simulink library "DiSC_ToolboxOpal_V12"  (R2012b)
settings: Solver=ode45  StartTime=0.0  StopTime=10.0  RelTol=1e-3
undefined symbols (not defined in the file or in its folder): SamplingTime
(part 4 of 5)

== matlab function DiSC_ToolboxOpal_V12/SuperMarket/MATLAB Function ==
  data: exeDefrost input; p output; pRS input; t input; q output; timeReady output; timeDefrost output
function [p,q,timeReady,timeDefrost] = smAssetDO(exeDefrost,pRS, t)
%#codegen
% Simulink version of supermarket model using embedded MATLAB function
%%Supermarket with flexible defrost cycles for demand response purpose
%   This class implements a model of a supermarket with flexible
%   defrost cycles. The defrost cycles of low temperature display cases
%   are allowed to be shifted in time under certain bounds. The reason
%   for only using low temperature dispaly cases is that these use
%   electrical heating elements for actively melting the ice during
%   defrost cycles. These heating elements consume a substantial amount
%   of power.
%
%   For a formal description of supermarket defrost flexibility, see the
%   note on the homepage:
%   http://kom.aau.dk/project/SmartGridControl/DiSC/documentation.html
%
% Revision:
% 16-07-2014, R. Pedersen, Aalborg University. Notes:
% 29-11-2014, R. Olsen/M. Kemal, Aalborg University (Simulink)
% 20-06-2015, F. Iov/M. Kemal, Aalborg University (Simulink toolbox for OPAL)

            % Implement algorithm. Calculate y as a function of
            % input u and discrete states.
             % Input:
            %   - exeDefrost [-], is the external control signal to execute defrost cycles.
            %   - pRS [W], is the power consumption of the refrigeration system, this should be provided as data.
            %
            % Output:
            %   - p [W], is the active power consumption of the supermarket.
            %   - q [VAR], is the reactive power consumption of the supermarket.
            %   - timeReady [s], is the time until defrost cycles are ready to be executed.
            %   - timeDefrost [s], is the time until the defrost cycles will be executed by the supermarket.
            
            % Power and time flexibility from defrost cycle


    % parameter properties
        param.sBase = 3e6;            % Complex power base [VA]. 
        param.Ts = 1;                 % Sampling time [sec]. 
        param.onPU = false;           % Indicates if the supermarket is used to simulate a system on per unit basis. true = yes, false = no [-]. 
        param.numDF = 2;              % Number of low temperature display cases [-]. 
        param.PF = 0.95;              % Power factor [-].
        param.pDefrost=[3e3 10e3];    % Vector containing defrost power consumption [W]. 
        
     persistent var;
     if isempty(var) 
        var.p_c=0;      %All used for caching in between sampling period
        var.q_c=0;
        var.tr_c=zeros(2,1);
        var.tdf_c=zeros(2,1);
        var.t_c=0;         
         
         
        var.readyTimers = zeros(2,1);
        var.defrostTimers = zeros(2,1);
        var.waitTimers = ones(2,1)*60*60*3;
        
        var.timeReady=zeros(2,1);  
        var.timeDefrost=zeros(2,1);
        var.waitGuards = ones(2,1)*60*60*10;      
        var.states = ones(2,1)*2;               
        var.readyGuards = ones(2,1)*60*60*2;    
        var.defrostGuards = ones(2,1)*45*60;    
        var.pVec =zeros(2,1);           
     end    
     
     %implement algorithm
            if (param.Ts>0)
               if (t>(var.t_c+param.Ts))
                   [p,q,timeReady,timeDefrost,varNew] = sampleSM(param,var,exeDefrost,pRS);
                   var=varNew;
                   var.p_c=p;
                   var.q_c=q;
                   var.tr_c=timeReady;
                   var.tdf_c=timeDefrost;
                   var.t_c=t;
               end
               p=var.p_c;
               q=var.q_c;
               timeReady=var.tr_c;
               timeDefrost=var.tdf_c;               
            else
                [p,q,timeReady,timeDefrost,varNew] = sampleSM(param,var,exeDefrost,pRS);
                var= varNew;
            end

end

== matlab function DiSC_ToolboxOpal_V12/Tap Changer/MATLAB Function ==
  data: y1 output; vMeas input; vRef input; uRef input; mode input; day input; y2 output; y3 output; time input
function [y1,y2,y3] = tcAssetDO(vMeas,vRef,uRef,mode,day,time)
%#codegen
   %tcAssetDO implements a controllable tap changing transformer using
   %MATLAB embedded block of simulink 
   %
   %
    %   The tcAsset can change the tap position of a transformer and 
    %   thereby effectively change the transformers ratio.
    %   The tap changer can be used to simulate e.g., an on-load tap changing
    %   transformer. The tap changer works by altering the grid admittance
    %   matrix, when ever the tap position is changed. To ensure realistic
    %   simulation scenarios a minimum time between tap changes has been
    %   incorporated, along with a specified maximum number of tap changes
    %   per day.
    %   
    %   The model is intended for studing voltage control problems and can
    %   be set to run in two different modes; follow tap reference and
    %   apply voltage control. The model is based on the one found in "Power Systems
    %   Stability and Control, P. Kundur".
    %
    % Revision:
    % 03-09-2014, R. Pedersen, Aalborg University. Notes:
    % 29-11-2014, R. Olsen/M. Kemal, Aalborg University (Simulink)
    % 20-06-2015, F. Iov/M. Kemal, Aalborg University (Simulink toolbox for OPAL)
            % Input:
            %   - v, is the voltage at the connection point.
            %   - vRef, is the voltage reference for the voltage
            %     control.
            %   - uRef, is the reference to tap position.
            %   - k, is the sample.
            %   - day, is the day of the simulation (1-365).
            % 
            % Output:
            %   - y1, y2, y3, is the transformer admittances between busses,
            %     from ground to primary side bus and from ground to
            %     secondary side bus, respectively.    
    %parameter properties
        param.vBase = 20e3;               % Voltage base [V].
        param.Z = 0.03-0.13i;             % Trafo impedance [Ohm].
        param.Ts = 1;                     % Sampling time [sec].
        param.nomTapRatio = 3;            % Nominal transformer ratio [-].
        param.nTapUp = 5;                 % Number of tap position upwards [-].
        param.nTapDown = -5;              % Number of tap positions downwards [-].
        param.nTapPrDay = 10;             % Maximum number of tap changes per day [-].
        param.chPrTap = 0.0125;           % Ratio of change from nominal voltage per tap position on a per unit basis [-].
        param.tMin = 5*60;                % Minimum time between tap changes [sec]. 

    %variable properties     
     persistent var;
     if isempty(var) 
        % Setup the buffer for the moving average filter
        %vAvgFilterTemp=1;
        var.avgFilterBuf = ones(10,1);  %TODO: This has been static defined due to Simulink
        var.kMin=0 ;                       % [-]. Minimum number of samples between tap changes
        
        var.tapChOk = 0;                % [-]. Flag indicating if tap change is allowed (1=yes, 0=no) 
        var.y1 = complex(0);            % [S]. Admittance of trafo between busses
        var.y2 = complex(0);            % [S]. Admittance from ground to trafo, primary side
        var.y3 = complex(0);            % [S]. Admittance from ground to trafo, secondary side
        var.tapPos = -1;                % [-]. Tap position
        var.dayOld = -1;                % [-]. Used to check if day has changed
        var.tapChDay = 0;               % [-]. Number of tap changes that has occured in a day
        var.tapTimer = 0;               % [-]. Timer indicating if tap changing is allowed, i.e., the timer must be greater than kMin to do tap changing
        var.vHyst = 0.05;               % [%]. Hysterisis limit for voltage control
        var.avgFilterTime = 10*60;      % [s]. Time window of the moving average filter
        var.mode = 0;                   % [-]. Mode of the tap position control (0=follow tap reference, 1=voltage control
        var.t_c=0;                      % [s]. Caching time
        var.y1_c=complex(0);            % Cached y1 value
        var.y2_c=complex(0);
        var.y3_c=complex(0);
        var.k=0;                        % Sample nr.         
     end
            % Compute minimum samples between tap changes
            var.kMin = ceil(param.tMin/param.Ts);
            
            % Change the admittances of the trafo
            [var.y1_c,var.y2_c,var.y3_c] = sampletcAsset(param,var,1,1,0,1,1);
            var.tapTimer = 0;
            var.tapChDay = 0;
            var.tapChOk = 0;
            %changeTrafoAdm(obj); 
            
            % Set average filter buffer
            var.avgFilterBuf = var.avgFilterBuf*param.vBase;
            
                        % Implement algorithm. 
           
             if (param.Ts>0)
               if (time>(var.t_c+param.Ts))
                   [y1,y2,y3,varNew] = sampletcAsset(param,var,vMeas,vRef,uRef,var.k,day);
                   var=varNew;
                   var.y1_c=y1;
                   var.y2_c=y2;
                   var.y3_c=y3;
                   var.t_c=time;
                   var.k=var.k+1;
                   var.mode = mode;
               end
               y1=var.y1_c;
               y2=var.y2_c;
               y3=var.y3_c;               
            else
                [y1,y2,y3,varNew] = sampletcAsset(param,var,vMeas,vRef,uRef,var.k,day);
                var=varNew;
                var.k=var.k+1; 
             end     
                
end

== matlab function DiSC_ToolboxOpal_V12/SolarPowerPlantDO/pvAssetDO/MATLAB Function1 ==
  data: solarIrr input; p output; vMeas input; time input; dP input; dPlim input; qRef input; qMode input; vRef input; q output; pAva output
function [p,q,pAva] = pvAssetDO(solarIrr,vMeas,time,dP,dPlim,qRef,qMode,vRef)

%#codegen
%pvAssetDO implements a simple P,Q controllable solar PV system using MATLAB embedded function.
    %   The pvAsset can be set to follow an active power reference, output
    %   maximum power available or derate power. It can also, at the same
    %   time be set to follow a reactive power reference, output the
    %   minimum reactive power according to the power factor or try to keep
    %   a voltage reference in the coupling point by controlling reactive
    %   power output.
    %   
    %   
    % Revision:
    % 19-06-2014, R. Pedersen, Aalborg University. Notes:
    % R. Pedersen 11-6-2014, Aalborg University
    % 29-11-2014, R. Olsen/M. Kemal, Aalborg University (Simulink)
    % 20-06-2015, F. Iov/M. Kemal, Aalborg University (Simulink toolbox for OPAL)
    
                % Input:
            %   - s [w/m^2], is the solar irradiance.
            %   - v [V], is the voltage at the connection point.
            %   - dP [PU], is the reference to active power change (curtailment).
            %   - dPlim [PU], is the reference to derated power (derate)
            %   - qRef [VAR], is the reactive power reference.
            %   - vRef [V], is the voltage reference.
            %
            % Output:
            %   - p [W], is the active power output
            %   - q [VAR], is the reactive power output
            %   - pAva [W], is the available power

            
           
        %properties
        param.vBase = 400;                % Voltage base [V].
        param.pRated = 6e3;               % Rated output power [W].
        param.sMax = 6e3;                 % Maximum apparent power [VA].
        param.A = 25;                     % Area of PV cell [m^2].
        param.eta = 0.25;                  % Efficency of cell [-].
        param.PF = 1;                     % Power factor [-].
        param.Ts = 60;                    % Sampling time (set to 0 if not used)

     %variable properties     
     persistent var;
     if isempty(var) 
        var.t_c = 0;                    %Time of caching
        var.p_c = 0;                    %Cached values
        var.q_c = 0;
        var.pAva_c = 0;
        var.kPV = 0;               % Gain from s to p [-].
        var.Qmode = 0;                  % Reactive power control mode [-].         
     end

        
        
% Solar to power conversion factor
     var.kPV = param.eta*param.A;
     
           if (param.Ts>0)
               if (time>(var.t_c+param.Ts))
                   [p,q,pAva,varNew] = samplePV(param,var,solarIrr,vMeas,dP,dPlim,qRef,vRef);
                   var=varNew;
                   var.p_c=p;
                   var.q_c=q;
                   var.pAva_c=pAva;
                   var.t_c=time;
                   var.Qmode = qMode;
               end
               p=var.p_c;
               q=var.q_c;
               pAva=var.pAva_c;
            else
               [p,q,pAva,varNew] = samplePV(param,var,solarIrr,vMeas,dP,dPlim,qRef,vRef);
               var=varNew;
               var.Qmode = qMode;
            end    

    
    
            
  end

== matlab function DiSC_ToolboxOpal_V12/SolarPowerPlantDO/pvAssetDO1/MATLAB Function1 ==
  data: solarIrr input; p output; vMeas input; time input; dP input; dPlim input; qRef input; qMode input; vRef input; q output; pAva output
function [p,q,pAva] = pvAssetDO(solarIrr,vMeas,time,dP,dPlim,qRef,qMode,vRef)

%#codegen
%pvAssetDO implements a simple P,Q controllable solar PV system using MATLAB embedded function.
    %   The pvAsset can be set to follow an active power reference, output
    %   maximum power available or derate power. It can also, at the same
    %   time be set to follow a reactive power reference, output the
    %   minimum reactive power according to the power factor or try to keep
    %   a voltage reference in the coupling point by controlling reactive
    %   power output.
    %   
    %   
    % Revision:
    % 19-06-2014, R. Pedersen, Aalborg University. Notes:
    % R. Pedersen 11-6-2014, Aalborg University
    % 29-11-2014, R. Olsen/M. Kemal, Aalborg University (Simulink)
    % 20-06-2015, F. Iov/M. Kemal, Aalborg University (Simulink toolbox for OPAL)
    
                % Input:
            %   - s [w/m^2], is the solar irradiance.
            %   - v [V], is the voltage at the connection point.
            %   - dP [PU], is the reference to active power change (curtailment).
            %   - dPlim [PU], is the reference to derated power (derate)
            %   - qRef [VAR], is the reactive power reference.
            %   - vRef [V], is the voltage reference.
            %
            % Output:
            %   - p [W], is the active power output
            %   - q [VAR], is the reactive power output
            %   - pAva [W], is the available power

            
           
        %properties
        param.vBase = 400;                % Voltage base [V].
        param.pRated = 6e3;               % Rated output power [W].
        param.sMax = 6e3;                 % Maximum apparent power [VA].
        param.A = 25;                     % Area of PV cell [m^2].
        param.eta = 0.25;                  % Efficency of cell [-].
        param.PF = 1;                     % Power factor [-].
        param.Ts = 60;                    % Sampling time (set to 0 if not used)

     %variable properties     
     persistent var;
     if isempty(var) 
        var.t_c = 0;                    %Time of caching
        var.p_c = 0;                    %Cached values
        var.q_c = 0;
        var.pAva_c = 0;
        var.kPV = 0;               % Gain from s to p [-].
        var.Qmode = 0;                  % Reactive power control mode [-].         
     end

        
        
% Solar to power conversion factor
     var.kPV = param.eta*param.A;
     
           if (param.Ts>0)
               if (time>(var.t_c+param.Ts))
                   [p,q,pAva,varNew] = samplePV(param,var,solarIrr,vMeas,dP,dPlim,qRef,vRef);
                   var=varNew;
                   var.p_c=p;
                   var.q_c=q;
                   var.pAva_c=pAva;
                   var.t_c=time;
                   var.Qmode = qMode;
               end
               p=var.p_c;
               q=var.q_c;
               pAva=var.pAva_c;
            else
               [p,q,pAva,varNew] = samplePV(param,var,solarIrr,vMeas,dP,dPlim,qRef,vRef);
               var=varNew;
               var.Qmode = qMode;
            end    

    
    
            
  end

== matlab function DiSC_ToolboxOpal_V12/SolarPowerPlantDO/pvAssetDO2/MATLAB Function1 ==
  data: solarIrr input; p output; vMeas input; time input; dP input; dPlim input; qRef input; qMode input; vRef input; q output; pAva output
function [p,q,pAva] = pvAssetDO(solarIrr,vMeas,time,dP,dPlim,qRef,qMode,vRef)

%#codegen
%pvAssetDO implements a simple P,Q controllable solar PV system using MATLAB embedded function.
    %   The pvAsset can be set to follow an active power reference, output
    %   maximum power available or derate power. It can also, at the same
    %   time be set to follow a reactive power reference, output the
    %   minimum reactive power according to the power factor or try to keep
    %   a voltage reference in the coupling point by controlling reactive
    %   power output.
    %   
    %   
    % Revision:
    % 19-06-2014, R. Pedersen, Aalborg University. Notes:
    % R. Pedersen 11-6-2014, Aalborg University
    % 29-11-2014, R. Olsen/M. Kemal, Aalborg University (Simulink)
    % 20-06-2015, F. Iov/M. Kemal, Aalborg University (Simulink toolbox for OPAL)
    
                % Input:
            %   - s [w/m^2], is the solar irradiance.
            %   - v [V], is the voltage at the connection point.
            %   - dP [PU], is the reference to active power change (curtailment).
            %   - dPlim [PU], is the reference to derated power (derate)
            %   - qRef [VAR], is the reactive power reference.
            %   - vRef [V], is the voltage reference.
            %
            % Output:
            %   - p [W], is the active power output
            %   - q [VAR], is the reactive power output
            %   - pAva [W], is the available power

            
           
        %properties
        param.vBase = 400;                % Voltage base [V].
        param.pRated = 6e3;               % Rated output power [W].
        param.sMax = 6e3;                 % Maximum apparent power [VA].
        param.A = 25;                     % Area of PV cell [m^2].
        param.eta = 0.25;                  % Efficency of cell [-].
        param.PF = 1;                     % Power factor [-].
        param.Ts = 60;                    % Sampling time (set to 0 if not used)

     %variable properties     
     persistent var;
     if isempty(var) 
        var.t_c = 0;                    %Time of caching
        var.p_c = 0;                    %Cached values
        var.q_c = 0;
        var.pAva_c = 0;
        var.kPV = 0;               % Gain from s to p [-].
        var.Qmode = 0;                  % Reactive power control mode [-].         
     end

        
        
% Solar to power conversion factor
     var.kPV = param.eta*param.A;
     
           if (param.Ts>0)
               if (time>(var.t_c+param.Ts))
                   [p,q,pAva,varNew] = samplePV(param,var,solarIrr,vMeas,dP,dPlim,qRef,vRef);
                   var=varNew;
                   var.p_c=p;
                   var.q_c=q;
                   var.pAva_c=pAva;
                   var.t_c=time;
                   var.Qmode = qMode;
               end
               p=var.p_c;
               q=var.q_c;
               pAva=var.pAva_c;
            else
               [p,q,pAva,varNew] = samplePV(param,var,solarIrr,vMeas,dP,dPlim,qRef,vRef);
               var=varNew;
               var.Qmode = qMode;
            end    

    
    
            
  end

== matlab function DiSC_ToolboxOpal_V12/SolarPowerPlantDO/pvAssetDO3/MATLAB Function1 ==
  data: solarIrr input; p output; vMeas input; time input; dP input; dPlim input; qRef input; qMode input; vRef input; q output; pAva output
function [p,q,pAva] = pvAssetDO(solarIrr,vMeas,time,dP,dPlim,qRef,qMode,vRef)

%#codegen
%pvAssetDO implements a simple P,Q controllable solar PV system using MATLAB embedded function.
    %   The pvAsset can be set to follow an active power reference, output
    %   maximum power available or derate power. It can also, at the same
    %   time be set to follow a reactive power reference, output the
    %   minimum reactive power according to the power factor or try to keep
    %   a voltage reference in the coupling point by controlling reactive
    %   power output.
    %   
    %   
    % Revision:
    % 19-06-2014, R. Pedersen, Aalborg University. Notes:
    % R. Pedersen 11-6-2014, Aalborg University
    % 29-11-2014, R. Olsen/M. Kemal, Aalborg University (Simulink)
    % 20-06-2015, F. Iov/M. Kemal, Aalborg University (Simulink toolbox for OPAL)
    
                % Input:
            %   - s [w/m^2], is the solar irradiance.
            %   - v [V], is the voltage at the connection point.
            %   - dP [PU], is the reference to active power change (curtailment).
            %   - dPlim [PU], is the reference to derated power (derate)
            %   - qRef [VAR], is the reactive power reference.
            %   - vRef [V], is the voltage reference.
            %
            % Output:
            %   - p [W], is the active power output
            %   - q [VAR], is the reactive power output
            %   - pAva [W], is the available power

            
           
        %properties
        param.vBase = 400;                % Voltage base [V].
        param.pRated = 6e3;               % Rated output power [W].
        param.sMax = 6e3;                 % Maximum apparent power [VA].
        param.A = 25;                     % Area of PV cell [m^2].
        param.eta = 0.25;                  % Efficency of cell [-].
        param.PF = 1;                     % Power factor [-].
        param.Ts = 60;                    % Sampling time (set to 0 if not used)

     %variable properties     
     persistent var;
     if isempty(var) 
        var.t_c = 0;                    %Time of caching
        var.p_c = 0;                    %Cached values
        var.q_c = 0;
        var.pAva_c = 0;
        var.kPV = 0;               % Gain from s to p [-].
        var.Qmode = 0;                  % Reactive power control mode [-].         
     end

        
        
% Solar to power conversion factor
     var.kPV = param.eta*param.A;
     
           if (param.Ts>0)
               if (time>(var.t_c+param.Ts))
                   [p,q,pAva,varNew] = samplePV(param,var,solarIrr,vMeas,dP,dPlim,qRef,vRef);
                   var=varNew;
                   var.p_c=p;
                   var.q_c=q;
                   var.pAva_c=pAva;
                   var.t_c=time;
                   var.Qmode = qMode;
               end
               p=var.p_c;
               q=var.q_c;
               pAva=var.pAva_c;
            else
               [p,q,pAva,varNew] = samplePV(param,var,solarIrr,vMeas,dP,dPlim,qRef,vRef);
               var=varNew;
               var.Qmode = qMode;
            end    

    
    
            
  end

== matlab function DiSC_ToolboxOpal_V12/SolarPowerPlantDO/pvAssetDO4/MATLAB Function1 ==
  data: solarIrr input; p output; vMeas input; time input; dP input; dPlim input; qRef input; qMode input; vRef input; q output; pAva output
function [p,q,pAva] = pvAssetDO(solarIrr,vMeas,time,dP,dPlim,qRef,qMode,vRef)

%#codegen
%pvAssetDO implements a simple P,Q controllable solar PV system using MATLAB embedded function.
    %   The pvAsset can be set to follow an active power reference, output
    %   maximum power available or derate power. It can also, at the same
    %   time be set to follow a reactive power reference, output the
    %   minimum reactive power according to the power factor or try to keep
    %   a voltage reference in the coupling point by controlling reactive
    %   power output.
    %   
    %   
    % Revision:
    % 19-06-2014, R. Pedersen, Aalborg University. Notes:
    % R. Pedersen 11-6-2014, Aalborg University
    % 29-11-2014, R. Olsen/M. Kemal, Aalborg University (Simulink)
    % 20-06-2015, F. Iov/M. Kemal, Aalborg University (Simulink toolbox for OPAL)
    
                % Input:
            %   - s [w/m^2], is the solar irradiance.
            %   - v [V], is the voltage at the connection point.
            %   - dP [PU], is the reference to active power change (curtailment).
            %   - dPlim [PU], is the reference to derated power (derate)
            %   - qRef [VAR], is the reactive power reference.
            %   - vRef [V], is the voltage reference.
            %
            % Output:
            %   - p [W], is the active power output
            %   - q [VAR], is the reactive power output
            %   - pAva [W], is the available power

            
           
        %properties
        param.vBase = 400;                % Voltage base [V].
        param.pRated = 6e3;               % Rated output power [W].
        param.sMax = 6e3;                 % Maximum apparent power [VA].
        param.A = 25;                     % Area of PV cell [m^2].
        param.eta = 0.25;                  % Efficency of cell [-].
        param.PF = 1;                     % Power factor [-].
        param.Ts = 60;                    % Sampling time (set to 0 if not used)

     %variable properties     
     persistent var;
     if isempty(var) 
        var.t_c = 0;                    %Time of caching
        var.p_c = 0;                    %Cached values
        var.q_c = 0;
        var.pAva_c = 0;
        var.kPV = 0;               % Gain from s to p [-].
        var.Qmode = 0;                  % Reactive power control mode [-].         
     end

        
        
% Solar to power conversion factor
     var.kPV = param.eta*param.A;
     
           if (param.Ts>0)
               if (time>(var.t_c+param.Ts))
                   [p,q,pAva,varNew] = samplePV(param,var,solarIrr,vMeas,dP,dPlim,qRef,vRef);
                   var=varNew;
                   var.p_c=p;
                   var.q_c=q;
                   var.pAva_c=pAva;
                   var.t_c=time;
                   var.Qmode = qMode;
               end
               p=var.p_c;
               q=var.q_c;
               pAva=var.pAva_c;
            else
               [p,q,pAva,varNew] = samplePV(param,var,solarIrr,vMeas,dP,dPlim,qRef,vRef);
               var=varNew;
               var.Qmode = qMode;
            end    

    
    
            
  end

== matlab function DiSC_ToolboxOpal_V12/SolarPowerPlantDO/pvAssetDO5/MATLAB Function1 ==
  data: solarIrr input; p output; vMeas input; time input; dP input; dPlim input; qRef input; qMode input; vRef input; q output; pAva output
function [p,q,pAva] = pvAssetDO(solarIrr,vMeas,time,dP,dPlim,qRef,qMode,vRef)

%#codegen
%pvAssetDO implements a simple P,Q controllable solar PV system using MATLAB embedded function.
    %   The pvAsset can be set to follow an active power reference, output
    %   maximum power available or derate power. It can also, at the same
    %   time be set to follow a reactive power reference, output the
    %   minimum reactive power according to the power factor or try to keep
    %   a voltage reference in the coupling point by controlling reactive
    %   power output.
    %   
    %   
    % Revision:
    % 19-06-2014, R. Pedersen, Aalborg University. Notes:
    % R. Pedersen 11-6-2014, Aalborg University
    % 29-11-2014, R. Olsen/M. Kemal, Aalborg University (Simulink)
    % 20-06-2015, F. Iov/M. Kemal, Aalborg University (Simulink toolbox for OPAL)
    
                % Input:
            %   - s [w/m^2], is the solar irradiance.
            %   - v [V], is the voltage at the connection point.
            %   - dP [PU], is the reference to active power change (curtailment).
            %   - dPlim [PU], is the reference to derated power (derate)
            %   - qRef [VAR], is the reactive power reference.
            %   - vRef [V], is the voltage reference.
            %
            % Output:
            %   - p [W], is the active power output
            %   - q [VAR], is the reactive power output
            %   - pAva [W], is the available power

            
           
        %properties
        param.vBase = 400;                % Voltage base [V].
        param.pRated = 6e3;               % Rated output power [W].
        param.sMax = 6e3;                 % Maximum apparent power [VA].
        param.A = 25;                     % Area of PV cell [m^2].
        param.eta = 0.25;                  % Efficency of cell [-].
        param.PF = 1;                     % Power factor [-].
        param.Ts = 60;                    % Sampling time (set to 0 if not used)

     %variable properties     
     persistent var;
     if isempty(var) 
        var.t_c = 0;                    %Time of caching
        var.p_c = 0;                    %Cached values
        var.q_c = 0;
        var.pAva_c = 0;
        var.kPV = 0;               % Gain from s to p [-].
        var.Qmode = 0;                  % Reactive power control mode [-].         
     end

        
        
% Solar to power conversion factor
     var.kPV = param.eta*param.A;
     
           if (param.Ts>0)
               if (time>(var.t_c+param.Ts))
                   [p,q,pAva,varNew] = samplePV(param,var,solarIrr,vMeas,dP,dPlim,qRef,vRef);
                   var=varNew;
                   var.p_c=p;
                   var.q_c=q;
                   var.pAva_c=pAva;
                   var.t_c=time;
                   var.Qmode = qMode;
               end
               p=var.p_c;
               q=var.q_c;
               pAva=var.pAva_c;
            else
               [p,q,pAva,varNew] = samplePV(param,var,solarIrr,vMeas,dP,dPlim,qRef,vRef);
               var=varNew;
               var.Qmode = qMode;
            end    

    
    
            
  end

== matlab function DiSC_ToolboxOpal_V12/WindPowerPlant/wtAssetDO/MATLAB Function ==
  data: p output; wind input; vMeas input; dP input; dPlim input; qRef input; qMode input; vRef input; time input; q output; pAva output
function [p,q,pAva] = wtAssetSDO(wind,vMeas,dP,dPlim,qRef,qMode,vRef, time)
%#codegen
    %wtAssetS implements a simple P,Q controllable wind turbine system for Simulink.
    % This model works for Simulink and requires generatedWindFiles to
    % have been executed before running the simulink model
    % 
    %   The wtAsset can be set to follow an active power reference, output
    %   maximum power available or curtail power. It can also, at the same
    %   time be set to follow a reactive power reference, output the
    %   minimum reactive power according to the power factor or try to keep
    %   a voltage reference in the coupling point by controlling reactive
    %   power output.
    %   
    %   The model is partly based on the book
    %   "Optimal Control of Wind Energy Systems 2008".
    %   
    %   
    % Revision:
    % 23-05-2014, C. E. Sloth and R. Pedersen, Aalborg University. Notes:
    % 29-11-2014, R. Olsen/M. Kemal, Aalborg University (Simulink)
         %Parameters
        param.vBase = 20e3;               % Voltage base [V].
        param.pRated = 100e3;               % Rated output power [W].
        param.sMax = 100e3;                 % Maximum apparent power [VA].
        param.wMin = 3;                   % Cut-in wind speed [m/s].
        param.wMax = 25;                  % Cut-out wind speed [m/s].
        param.wRated = 12;                % Rated wind speed [m/s].
        param.rfTau = 20;                 % Time constant of rotor filter [s].
        param.PF = 1;                     % Power factor [-].
        param.Ts = 60;                    % Sampling time [sec].  

     %variables 
     persistent var;
     if isempty(var)         
        var.p_c=0;                      %All used for caching in between sampling period
        var.q_c=0;
        var.pAva_c=0;
        var.t_c=0;
        var.pOld = 0;                   % [w]. Place holder for the rotor initia filter
        
        var.avgFilterTime = 10*60;      % [s]. Time that the filter should look back 
        var.avgFilterBuf = zeros(ceil(10*60/60),1);
        var.Qmode = 0;                  % [-]. Reactive power control mode
        var.kWT = 3e6/(12^3);           % [-]. Gain from w^3 to p
     end

            % Power conversion constant
            var.kWT = param.pRated/(param.wRated^3);    
            
            % Implement algorithm. 
            
            if (param.Ts>0)
               if (time>(var.t_c+param.Ts))
                   [p,q,pAva,varNew] = sampleWT(param,var,wind,vMeas,dP,dPlim,qRef,vRef);
                   varNew.p_c=p;
                   varNew.q_c=q;
                   varNew.pAva_c=pAva;
                   varNew.t_c=time;
                   varNew.Qmode = qMode;
                   var=varNew;
               end
               p=var.p_c;
               q=var.q_c;
               pAva=var.pAva_c;
            else
                [p,q,pAva,varNew] = sampleWT(param,var,wind,vMeas,dP,dPlim,qRef,vRef);
                var=varNew;
            end
            
        
            
%          [p,q,pAva,varNew] = sampleWT(obj,var,wind,vMeas,dP,dPlim,qRef,vRef);
         
         
end

== matlab function DiSC_ToolboxOpal_V12/WindPowerPlant/wtAssetDO1/MATLAB Function ==
  data: p output; wind input; vMeas input; dP input; dPlim input; qRef input; qMode input; vRef input; time input; q output; pAva output
function [p,q,pAva] = wtAssetSDO(wind,vMeas,dP,dPlim,qRef,qMode,vRef, time)
%#codegen
    %wtAssetS implements a simple P,Q controllable wind turbine system for Simulink.
    % This model works for Simulink and requires generatedWindFiles to
    % have been executed before running the simulink model
    % 
    %   The wtAsset can be set to follow an active power reference, output
    %   maximum power available or curtail power. It can also, at the same
    %   time be set to follow a reactive power reference, output the
    %   minimum reactive power according to the power factor or try to keep
    %   a voltage reference in the coupling point by controlling reactive
    %   power output.
    %   
    %   The model is partly based on the book
    %   "Optimal Control of Wind Energy Systems 2008".
    %   
    %   
    % Revision:
    % 23-05-2014, C. E. Sloth and R. Pedersen, Aalborg University. Notes:
    % 29-11-2014, R. Olsen/M. Kemal, Aalborg University (Simulink)
         %Parameters
        param.vBase = 20e3;               % Voltage base [V].
        param.pRated = 100e3;               % Rated output power [W].
        param.sMax = 100e3;                 % Maximum apparent power [VA].
        param.wMin = 3;                   % Cut-in wind speed [m/s].
        param.wMax = 25;                  % Cut-out wind speed [m/s].
        param.wRated = 12;                % Rated wind speed [m/s].
        param.rfTau = 20;                 % Time constant of rotor filter [s].
        param.PF = 1;                     % Power factor [-].
        param.Ts = 60;                    % Sampling time [sec].  

     %variables 
     persistent var;
     if isempty(var)         
        var.p_c=0;                      %All used for caching in between sampling period
        var.q_c=0;
        var.pAva_c=0;
        var.t_c=0;
        var.pOld = 0;                   % [w]. Place holder for the rotor initia filter
        
        var.avgFilterTime = 10*60;      % [s]. Time that the filter should look back 
        var.avgFilterBuf = zeros(ceil(10*60/60),1);
        var.Qmode = 0;                  % [-]. Reactive power control mode
        var.kWT = 3e6/(12^3);           % [-]. Gain from w^3 to p
     end

            % Power conversion constant
            var.kWT = param.pRated/(param.wRated^3);    
            
            % Implement algorithm. 
            
            if (param.Ts>0)
               if (time>(var.t_c+param.Ts))
                   [p,q,pAva,varNew] = sampleWT(param,var,wind,vMeas,dP,dPlim,qRef,vRef);
                   varNew.p_c=p;
                   varNew.q_c=q;
                   varNew.pAva_c=pAva;
                   varNew.t_c=time;
                   varNew.Qmode = qMode;
                   var=varNew;
               end
               p=var.p_c;
               q=var.q_c;
               pAva=var.pAva_c;
            else
                [p,q,pAva,varNew] = sampleWT(param,var,wind,vMeas,dP,dPlim,qRef,vRef);
                var=varNew;
            end
            
        
            
%          [p,q,pAva,varNew] = sampleWT(obj,var,wind,vMeas,dP,dPlim,qRef,vRef);
         
         
end

== matlab function DiSC_ToolboxOpal_V12/WindPowerPlant/wtAssetDO2/MATLAB Function ==
  data: p output; wind input; vMeas input; dP input; dPlim input; qRef input; qMode input; vRef input; time input; q output; pAva output
function [p,q,pAva] = wtAssetSDO(wind,vMeas,dP,dPlim,qRef,qMode,vRef, time)
%#codegen
    %wtAssetS implements a simple P,Q controllable wind turbine system for Simulink.
    % This model works for Simulink and requires generatedWindFiles to
    % have been executed before running the simulink model
    % 
    %   The wtAsset can be set to follow an active power reference, output
    %   maximum power available or curtail power. It can also, at the same
    %   time be set to follow a reactive power reference, output the
    %   minimum reactive power according to the power factor or try to keep
    %   a voltage reference in the coupling point by controlling reactive
    %   power output.
    %   
    %   The model is partly based on the book
    %   "Optimal Control of Wind Energy Systems 2008".
    %   
    %   
    % Revision:
    % 23-05-2014, C. E. Sloth and R. Pedersen, Aalborg University. Notes:
    % 29-11-2014, R. Olsen/M. Kemal, Aalborg University (Simulink)
         %Parameters
        param.vBase = 20e3;               % Voltage base [V].
        param.pRated = 100e3;               % Rated output power [W].
        param.sMax = 100e3;                 % Maximum apparent power [VA].
        param.wMin = 3;                   % Cut-in wind speed [m/s].
        param.wMax = 25;                  % Cut-out wind speed [m/s].
        param.wRated = 12;                % Rated wind speed [m/s].
        param.rfTau = 20;                 % Time constant of rotor filter [s].
        param.PF = 1;                     % Power factor [-].
        param.Ts = 60;                    % Sampling time [sec].  

     %variables 
     persistent var;
     if isempty(var)         
        var.p_c=0;                      %All used for caching in between sampling period
        var.q_c=0;
        var.pAva_c=0;
        var.t_c=0;
        var.pOld = 0;                   % [w]. Place holder for the rotor initia filter
        
        var.avgFilterTime = 10*60;      % [s]. Time that the filter should look back 
        var.avgFilterBuf = zeros(ceil(10*60/60),1);
        var.Qmode = 0;                  % [-]. Reactive power control mode
        var.kWT = 3e6/(12^3);           % [-]. Gain from w^3 to p
     end

            % Power conversion constant
            var.kWT = param.pRated/(param.wRated^3);    
            
            % Implement algorithm. 
            
            if (param.Ts>0)
               if (time>(var.t_c+param.Ts))
                   [p,q,pAva,varNew] = sampleWT(param,var,wind,vMeas,dP,dPlim,qRef,vRef);
                   varNew.p_c=p;
                   varNew.q_c=q;
                   varNew.pAva_c=pAva;
                   varNew.t_c=time;
                   varNew.Qmode = qMode;
                   var=varNew;
               end
               p=var.p_c;
               q=var.q_c;
               pAva=var.pAva_c;
            else
                [p,q,pAva,varNew] = sampleWT(param,var,wind,vMeas,dP,dPlim,qRef,vRef);
                var=varNew;
            end
            
        
            
%          [p,q,pAva,varNew] = sampleWT(obj,var,wind,vMeas,dP,dPlim,qRef,vRef);
         
         
end

== matlab function DiSC_ToolboxOpal_V12/WindPowerPlant/wtAssetDO3/MATLAB Function ==
  data: p output; wind input; vMeas input; dP input; dPlim input; qRef input; qMode input; vRef input; time input; q output; pAva output
function [p,q,pAva] = wtAssetSDO(wind,vMeas,dP,dPlim,qRef,qMode,vRef, time)
%#codegen
    %wtAssetS implements a simple P,Q controllable wind turbine system for Simulink.
    % This model works for Simulink and requires generatedWindFiles to
    % have been executed before running the simulink model
    % 
    %   The wtAsset can be set to follow an active power reference, output
    %   maximum power available or curtail power. It can also, at the same
    %   time be set to follow a reactive power reference, output the
    %   minimum reactive power according to the power factor or try to keep
    %   a voltage reference in the coupling point by controlling reactive
    %   power output.
    %   
    %   The model is partly based on the book
    %   "Optimal Control of Wind Energy Systems 2008".
    %   
    %   
    % Revision:
    % 23-05-2014, C. E. Sloth and R. Pedersen, Aalborg University. Notes:
    % 29-11-2014, R. Olsen/M. Kemal, Aalborg University (Simulink)
         %Parameters
        param.vBase = 20e3;               % Voltage base [V].
        param.pRated = 100e3;               % Rated output power [W].
        param.sMax = 100e3;                 % Maximum apparent power [VA].
        param.wMin = 3;                   % Cut-in wind speed [m/s].
        param.wMax = 25;                  % Cut-out wind speed [m/s].
        param.wRated = 12;                % Rated wind speed [m/s].
        param.rfTau = 20;                 % Time constant of rotor filter [s].
        param.PF = 1;                     % Power factor [-].
        param.Ts = 60;                    % Sampling time [sec].  

     %variables 
     persistent var;
     if isempty(var)         
        var.p_c=0;                      %All used for caching in between sampling period
        var.q_c=0;
        var.pAva_c=0;
        var.t_c=0;
        var.pOld = 0;                   % [w]. Place holder for the rotor initia filter
        
        var.avgFilterTime = 10*60;      % [s]. Time that the filter should look back 
        var.avgFilterBuf = zeros(ceil(10*60/60),1);
        var.Qmode = 0;                  % [-]. Reactive power control mode
        var.kWT = 3e6/(12^3);           % [-]. Gain from w^3 to p
     end

            % Power conversion constant
            var.kWT = param.pRated/(param.wRated^3);    
            
            % Implement algorithm. 
            
            if (param.Ts>0)
               if (time>(var.t_c+param.Ts))
                   [p,q,pAva,varNew] = sampleWT(param,var,wind,vMeas,dP,dPlim,qRef,vRef);
                   varNew.p_c=p;
                   varNew.q_c=q;
                   varNew.pAva_c=pAva;
                   varNew.t_c=time;
                   varNew.Qmode = qMode;
                   var=varNew;
               end
               p=var.p_c;
               q=var.q_c;
               pAva=var.pAva_c;
            else
                [p,q,pAva,varNew] = sampleWT(param,var,wind,vMeas,dP,dPlim,qRef,vRef);
                var=varNew;
            end
            
        
            
%          [p,q,pAva,varNew] = sampleWT(obj,var,wind,vMeas,dP,dPlim,qRef,vRef);
         
         
end

== matlab function DiSC_ToolboxOpal_V12/WindPowerPlant/wtAssetDO4/MATLAB Function ==
  data: p output; wind input; vMeas input; dP input; dPlim input; qRef input; qMode input; vRef input; time input; q output; pAva output
function [p,q,pAva] = wtAssetSDO(wind,vMeas,dP,dPlim,qRef,qMode,vRef, time)
%#codegen
    %wtAssetS implements a simple P,Q controllable wind turbine system for Simulink.
    % This model works for Simulink and requires generatedWindFiles to
    % have been executed before running the simulink model
    % 
    %   The wtAsset can be set to follow an active power reference, output
    %   maximum power available or curtail power. It can also, at the same
    %   time be set to follow a reactive power reference, output the
    %   minimum reactive power according to the power factor or try to keep
    %   a voltage reference in the coupling point by controlling reactive
    %   power output.
    %   
    %   The model is partly based on the book
    %   "Optimal Control of Wind Energy Systems 2008".
    %   
    %   
    % Revision:
    % 23-05-2014, C. E. Sloth and R. Pedersen, Aalborg University. Notes:
    % 29-11-2014, R. Olsen/M. Kemal, Aalborg University (Simulink)
         %Parameters
        param.vBase = 20e3;               % Voltage base [V].
        param.pRated = 100e3;               % Rated output power [W].
        param.sMax = 100e3;                 % Maximum apparent power [VA].
        param.wMin = 3;                   % Cut-in wind speed [m/s].
        param.wMax = 25;                  % Cut-out wind speed [m/s].
        param.wRated = 12;                % Rated wind speed [m/s].
        param.rfTau = 20;                 % Time constant of rotor filter [s].
        param.PF = 1;                     % Power factor [-].
        param.Ts = 60;                    % Sampling time [sec].  

     %variables 
     persistent var;
     if isempty(var)         
        var.p_c=0;                      %All used for caching in between sampling period
        var.q_c=0;
        var.pAva_c=0;
        var.t_c=0;
        var.pOld = 0;                   % [w]. Place holder for the rotor initia filter
        
        var.avgFilterTime = 10*60;      % [s]. Time that the filter should look back 
        var.avgFilterBuf = zeros(ceil(10*60/60),1);
        var.Qmode = 0;                  % [-]. Reactive power control mode
        var.kWT = 3e6/(12^3);           % [-]. Gain from w^3 to p
     end

            % Power conversion constant
            var.kWT = param.pRated/(param.wRated^3);    
            
            % Implement algorithm. 
            
            if (param.Ts>0)
               if (time>(var.t_c+param.Ts))
                   [p,q,pAva,varNew] = sampleWT(param,var,wind,vMeas,dP,dPlim,qRef,vRef);
                   varNew.p_c=p;
                   varNew.q_c=q;
                   varNew.pAva_c=pAva;
                   varNew.t_c=time;
                   varNew.Qmode = qMode;
                   var=varNew;
               end
               p=var.p_c;
               q=var.q_c;
               pAva=var.pAva_c;
            else
                [p,q,pAva,varNew] = sampleWT(param,var,wind,vMeas,dP,dPlim,qRef,vRef);
                var=varNew;
            end
            
        
            
%          [p,q,pAva,varNew] = sampleWT(obj,var,wind,vMeas,dP,dPlim,qRef,vRef);
         
         
end
